simulink model "motor_pid_simulin"  (R2025a)
settings: Solver=VariableStepAuto  StartTime=0.0  StopTime=200  RelTol=1e-3
settings Model: Creator=JunfengWei  LastModifiedBy=JunfengWei

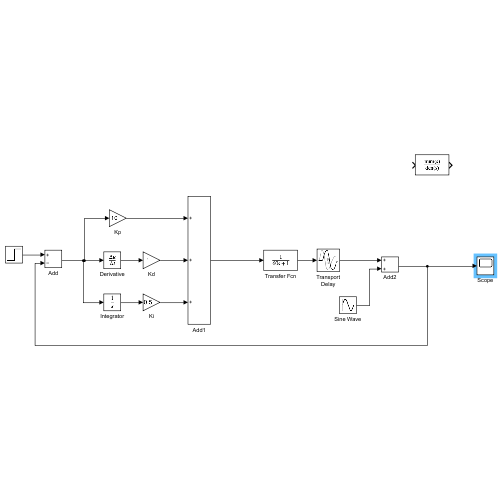
[thumbnail: Simulink's stored preview of the top-level diagram]
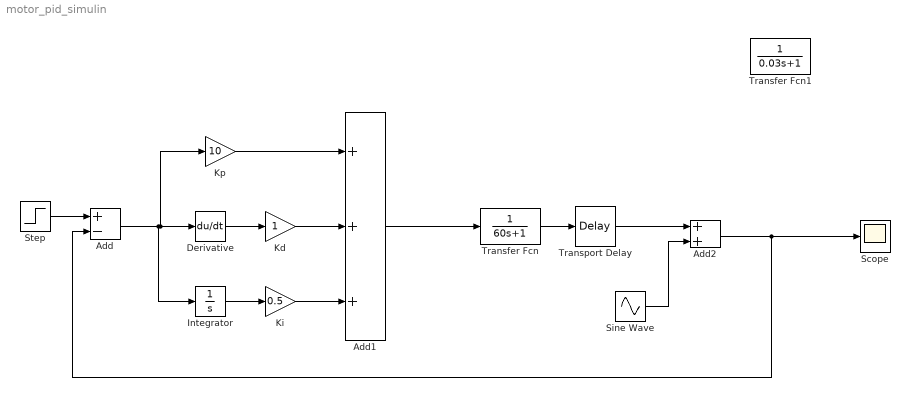
== system motor_pid_simulin ==
  Add : Sum  Inputs=+-
  Add1 : Sum  Inputs=+++
  Add2 : Sum
  Derivative : Derivative
  Integrator : Integrator
  Kd : Gain
  Ki : Gain  Gain=0.5
  Kp : Gain  Gain=10
  Scope : Scope
      settings: ActiveDisplayYMinimum=-2748.1013161795458  ActiveDisplayYMaximum=5889.5797136811134
  Sine Wave : Sin  Amplitude=0  Frequency=0  SampleTime=0
  Step : Step  After=1000  SampleTime=0
  Transfer Fcn : TransferFcn  Denominator=[60 1]
  Transfer Fcn1 : TransferFcn  Denominator=[0.03 1]
  Transport Delay : TransportDelay  DelayTime=0.001
  wires:
  Step/1 -> Add/1
  Add/1 -> Derivative/1, Kp/1, Integrator/1
  Integrator/1 -> Ki/1
  Derivative/1 -> Kd/1
  Kp/1 -> Add1/1
  Add1/1 -> Transfer Fcn/1
  Transfer Fcn/1 -> Transport Delay/1
  Transport Delay/1 -> Add2/1
  Kd/1 -> Add1/2
  Ki/1 -> Add1/3
  Sine Wave/1 -> Add2/2
  Add2/1 -> Scope/1, Add/2
